simulink model "sysp1"  (R2023a)
settings: Solver=VariableStepAuto  StartTime=0.0  StopTime=10.0  RelTol=1e-3
libraries: simulink x1
settings Model: Creator=miros  LastModifiedBy=miros
settings DebuggingCC: AlgebraicLoopMsg=none  ArtificialAlgebraicLoopMsg=none  MaxConsecutiveZCsMsg=none  ModelReferenceExtraNoncontSigs=none  OperatingPointInterfaceChecksumMismatchMsg=none

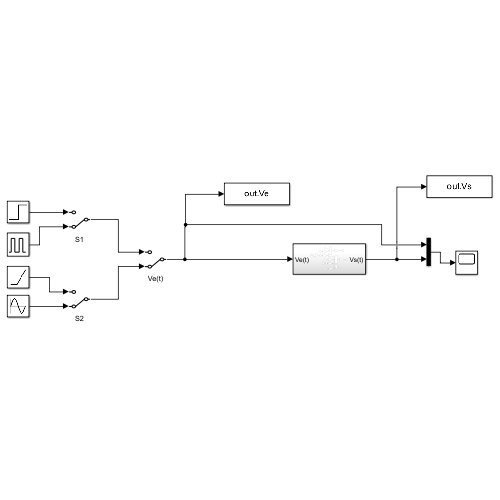
[thumbnail: Simulink's stored preview of the top-level diagram]
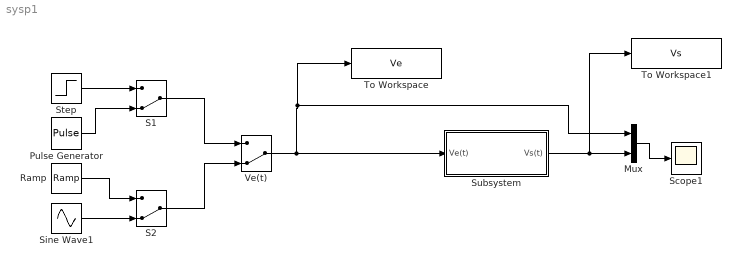
== system sysp1 ==
  Mux : Mux  Inputs=2
  Pulse Generator : DiscretePulseGenerator  PulseType=Time based  Period=10  PulseWidth=10  PhaseDelay=1
  Ramp : simulink/Sources/Ramp  slope=1/10  start=0  InitialOutput=0
  S1 : ManualSwitch  CurrentSetting=0
  S2 : ManualSwitch  CurrentSetting=0
  Scope1 : Scope
  Sine Wave1 : Sin  Frequency=pi/2  SampleTime=0
  Step : Step  Time=0  Before=1  SampleTime=0.001
  Subsystem : Subsystem
  To Workspace : ToWorkspace  VariableName=Ve  SampleTime=-1
  To Workspace1 : ToWorkspace  VariableName=Vs  SampleTime=-1
  Ve(t) : ManualSwitch  CurrentSetting=0
  wires:
  S2/1 -> Ve(t)/2
  Sine Wave1/1 -> S2/2
  Pulse Generator/1 -> S1/2
  Ramp/1 -> S2/1
  Step/1 -> S1/1
  S1/1 -> Ve(t)/1
  Ve(t)/1 -> Subsystem/1(Ve(t)), To Workspace/1, Mux/1
  Subsystem/1(Vs(t)) -> To Workspace1/1, Mux/2
  Mux/1 -> Scope1/1

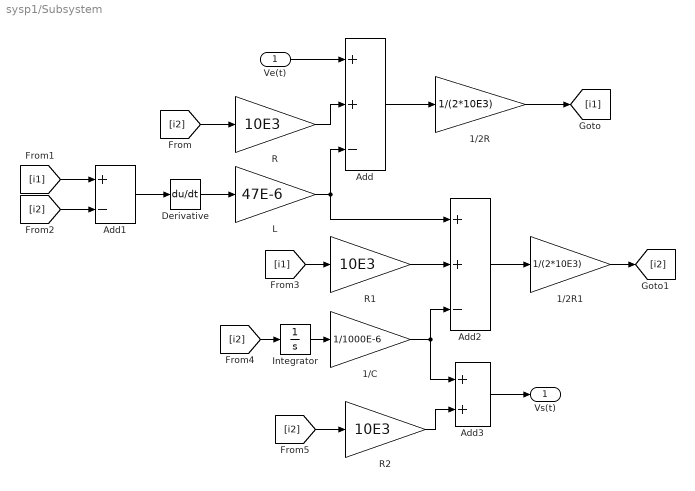
== system sysp1/Subsystem ==
  Ve(t) : Inport
  1/2R : Gain  Gain=1/(2*10E3)
  1/2R1 : Gain  Gain=1/(2*10E3)
  1/C : Gain  Gain=1/1000E-6
  Add : Sum  Inputs=++-
  Add1 : Sum  Inputs=+-
  Add2 : Sum  Inputs=++-
  Add3 : Sum
  Derivative : Derivative
  Integrator : Integrator
  L : Gain  Gain=47E-6
  R : Gain  Gain=10E3
  R1 : Gain  Gain=10E3
  R2 : Gain  Gain=10E3
  Vs(t) : Outport
  wires:
  Add2/1 -> 1/2R1/1
  1/2R1/1 -> [i2]
  Integrator/1 -> 1/C/1
  Add1/1 -> Derivative/1
  [i2] -> R/1
  [i2] -> R2/1
  Derivative/1 -> L/1
  Add/1 -> 1/2R/1
  R2/1 -> Add3/2
  L/1 -> Add2/1, Add/3
  R/1 -> Add/2
  [i2] -> Integrator/1
  [i2] -> Add1/2
  [i1] -> R1/1
  R1/1 -> Add2/2
  1/C/1 -> Add3/1, Add2/3
  [i1] -> Add1/1
  1/2R/1 -> [i1]
  Ve(t)/1 -> Add/1
  Add3/1 -> Vs(t)/1
